simulink model "finalcode"  (R2020a)
settings: Solver=FixedStepDiscrete  StartTime=0.0  StopTime=1  FixedStep=0.0005  RelTol=1e-3  EnableMultiTasking=on
undefined symbols (not defined in the file): acc_calmax1, acc_calmax2, acc_calmin1, acc_calmin2, akemancanshu, angle_middle, bre, bre_calmax, bre_calmin, chasuniujvvvv_hou, chasuniujvvvv_qian, chasuuuu, ecucoder_acal, I_AN01_5K1, I_AN03_5V, I_AN04_5V, kd, kddd, ki, kiii, kp, kppp, leftmax, O_SW06_HS1A, P11111, P22222, PIDmodel, PPPP, rightmax, slip, slip_big, slip_little, slipmodel, T_add, T_del, tiaoshi, TTTTTyouren, vvvv, zhiling
libraries: ec5744lib x305, canmsglib x97, simulink x23
(part 8 of 11)

== system finalcode/Subsystem/Tx/转向/检查模式转向/Subsystem/Subsystem ==
  Enable : EnablePort
  CAN Pack : canmsglib/CAN Pack  CANdbFile=C:\Users\Liu keliang\Desktop\HRT2023\HRT23赛季刘科良\CANdbc\steering.dbc  MsgList=(none)  MsgName=enable123  MsgIDType=Standard (11-bit identifier)  MsgIdentifier=291  MsgLength=1  Remote=off  ApplyMinMax=off  BusOutput=off  SignalInfo={'enable123','0','8','LE','unsigned','Standard','0','1','0','0','255'}
      settings: SourceProductBaseCode=ME,XP,VN  DataFormat=CANdb specified signals
  CAN Pack1 : canmsglib/CAN Pack  CANdbFile=C:\Users\Liu keliang\Desktop\HRT2023\HRT23赛季刘科良\CANdbc\steering.dbc  MsgList=(none)  MsgName=enable0  MsgIDType=Standard (11-bit identifier)  MsgIdentifier=0  MsgLength=8  Remote=off  ApplyMinMax=off  BusOutput=off  SignalInfo={'enable_00','0','16','LE','unsigned','Standard','0','1','0','0','65535';'enable_00_Copy_1','16','16','LE','unsigned','Standard','0','1','0','0','65535';'enable_00_Copy_2','32','16','LE','unsigned','Standard','0','1','0','0','65535';'enable_00_Copy_3','48','16','LE','unsigned','Standard','0','1','0','0','65535'}
      settings: SourceProductBaseCode=ME,XP,VN  DataFormat=CANdb specified signals
  CAN Pack2 : canmsglib/CAN Pack  CANdbFile=C:\Users\Liu keliang\Desktop\HRT2023\HRT23赛季刘科良\CANdbc\steering.dbc  MsgList=(none)  MsgName=enable401  MsgIDType=Standard (11-bit identifier)  MsgIdentifier=1025  MsgLength=6  Remote=off  ApplyMinMax=off  BusOutput=off  SignalInfo={'enable401','0','8','LE','unsigned','Standard','0','1','0','0','255';'enable401_Copy_1','8','8','LE','unsigned','Standard','0','1','0','0','255';'enable401_Copy_2','16','32','LE','signed','Standard','0','1','0','-2147483648','2147483647'}
      settings: SourceProductBaseCode=ME,XP,VN  DataFormat=CANdb specified signals
  CAN Pack4 : canmsglib/CAN Pack  CANdbFile=C:\Users\Liu keliang\Desktop\HRT2023\HRT23赛季刘科良\CANdbc\steering.dbc  MsgList=(none)  MsgName=enable80  MsgIDType=Standard (11-bit identifier)  MsgIdentifier=128  MsgLength=1  Remote=off  ApplyMinMax=off  BusOutput=off  SignalInfo={'dingshi','0','8','LE','unsigned','Standard','0','1','0','0','255'}
      settings: SourceProductBaseCode=ME,XP,VN  DataFormat=CANdb specified signals
  CANPackMessage : ec5744lib/RapidECU_U4B/04CANCommunication/CANPackMessage  datalength=1  sampletime=-1
      settings: SourceProductName=ECUCoder for MPC5744
  CANPackMessage1 : ec5744lib/RapidECU_U4B/04CANCommunication/CANPackMessage  datalength=8  sampletime=-1
      settings: SourceProductName=ECUCoder for MPC5744
  CANPackMessage2 : ec5744lib/RapidECU_U4B/04CANCommunication/CANPackMessage  datalength=6  sampletime=-1
      settings: SourceProductName=ECUCoder for MPC5744
  CANPackMessage4 : ec5744lib/RapidECU_U4B/04CANCommunication/CANPackMessage  datalength=1  sampletime=-1
      settings: SourceProductName=ECUCoder for MPC5744
  CANTransmit : ec5744lib/RapidECU_U4B/04CANCommunication/CANTransmit  canmodule=2  canbuffer=15  canmessageid=hex2dec('123')  canmessagetype=Standard(11-bit ID)  datalength=1  sampletime=-1
      settings: SourceProductName=ECUCoder for MPC5744
  CANTransmit1 : ec5744lib/RapidECU_U4B/04CANCommunication/CANTransmit  canmodule=2  canbuffer=56  canmessageid=hex2dec('00')  canmessagetype=Standard(11-bit ID)  datalength=8  sampletime=-1
      settings: SourceProductName=ECUCoder for MPC5744
  CANTransmit2 : ec5744lib/RapidECU_U4B/04CANCommunication/CANTransmit  canmodule=2  canbuffer=57  canmessageid=hex2dec('401')  canmessagetype=Standard(11-bit ID)  datalength=6  sampletime=-1
      settings: SourceProductName=ECUCoder for MPC5744
  CANTransmit4 : ec5744lib/RapidECU_U4B/04CANCommunication/CANTransmit  canmodule=2  canbuffer=58  canmessageid=hex2dec('80')  canmessagetype=Standard(11-bit ID)  datalength=1  sampletime=-1
      settings: SourceProductName=ECUCoder for MPC5744
  Constant : Constant  Value=0  SampleTime=-1
  Constant1 : Constant  SampleTime=-1
  Constant{2..4,6} (4 alike) : Constant  Value=0
  Constant5 : Constant  Value=0  SampleTime=-1
  Data Type Conversion{,1..2,4} (4 alike) : DataTypeConversion  OutDataTypeStr=uint8
  MATLAB Function : MATLAB Function  TreatAsAtomicUnit=on
  Saturation : Saturate  UpperLimit=758000  LowerLimit=605000
  Terminator{,1..2,4} (4 alike) : Terminator
  Zero-Order Hold{,1..4} (5 alike) : ZeroOrderHold  SampleTime=-1
  wires:
  CANTransmit/1 -> Terminator/1
  Zero-Order Hold2/1 -> CAN Pack1/3
  MATLAB Function/2(y) -> CAN Pack2/1
  CAN Pack1/1 -> CANPackMessage1/1
  CANTransmit2/1 -> Terminator2/1
  CANPackMessage4/1 -> Data Type Conversion4/1
  CAN Pack2/1 -> CANPackMessage2/1
  CANTransmit1/1 -> Terminator1/1
  Constant/1 -> Zero-Order Hold/1
  Data Type Conversion1/1 -> CANTransmit1/1
  Constant6/1 -> CAN Pack2/2
  CANTransmit4/1 -> Terminator4/1
  Data Type Conversion/1 -> CANTransmit/1
  Zero-Order Hold/1 -> CAN Pack/1
  CANPackMessage2/1 -> Data Type Conversion2/1
  CANPackMessage/1 -> Data Type Conversion/1
  Data Type Conversion4/1 -> CANTransmit4/1
  Constant4/1 -> Zero-Order Hold3/1
  CAN Pack/1 -> CANPackMessage/1
  CANPackMessage1/1 -> Data Type Conversion1/1
  Constant5/1 -> Zero-Order Hold4/1
  CAN Pack4/1 -> CANPackMessage4/1
  Constant3/1 -> Zero-Order Hold2/1
  Constant2/1 -> Zero-Order Hold1/1
  Constant1/1 -> CAN Pack1/1
  Zero-Order Hold4/1 -> CAN Pack4/1
  MATLAB Function/1(steer) -> Saturation/1
  Zero-Order Hold1/1 -> CAN Pack1/2
  Data Type Conversion2/1 -> CANTransmit2/1
  Zero-Order Hold3/1 -> CAN Pack1/4
  Saturation/1 -> CAN Pack2/3

== system finalcode/Subsystem/Tx/转向/检查模式转向/Subsystem/Subsystem1 ==
  y1 : Inport
  y2 : Inport  Port=2
  Enable : EnablePort
  CAN Pack5 : canmsglib/CAN Pack  CANdbFile=C:\Users\Liu keliang\Desktop\HRT2023\HRT23赛季刘科良\CANdbc\zhuanxiangresetting.dbc  MsgList=(none)  MsgName=reseting  MsgIDType=Standard (11-bit identifier)  MsgIdentifier=1537  MsgLength=8  Remote=off  ApplyMinMax=off  BusOutput=off  SignalInfo={'reseting1','0','32','LE','unsigned','Standard','0','1','0','-Inf','Inf';'reseting2','32','32','LE','unsigned','Standard','0','1','0','-Inf','Inf'}
      settings: SourceProductBaseCode=ME,XP,VN  DataFormat=CANdb specified signals
  CANPackMessage3 : ec5744lib/RapidECU_U4B/04CANCommunication/CANPackMessage  datalength=8  sampletime=-1
      settings: SourceProductName=ECUCoder for MPC5744
  CANTransmit3 : ec5744lib/RapidECU_U4B/04CANCommunication/CANTransmit  canmodule=2  canbuffer=61  canmessageid=hex2dec('601')  canmessagetype=Standard(11-bit ID)  datalength=8  sampletime=-1
      settings: SourceProductName=ECUCoder for MPC5744
  Data Type Conversion3 : DataTypeConversion  OutDataTypeStr=uint8
  Terminator3 : Terminator
  wires:
  CAN Pack5/1 -> CANPackMessage3/1
  y1/1 -> CAN Pack5/1
  CANTransmit3/1 -> Terminator3/1
  Data Type Conversion3/1 -> CANTransmit3/1
  CANPackMessage3/1 -> Data Type Conversion3/1
  y2/1 -> CAN Pack5/2

== system finalcode/Subsystem/Tx/转向/转向换算/Subsystem/integral ==
  Data Store Read12 : DataStoreRead  DataStoreName=zhuanjiaobianmaqi
  Data Store Read13 : DataStoreRead  DataStoreName=workstation_steering
  Sum of Elements : Sum  Inputs=+
  Sum1 : Sum  Inputs=|-+
  Tapped Delay : simulink/Discrete/Tapped Delay  vinit=0.0  samptime=-1  NumDelays=20  DelayOrder=Oldest  includeCurrent=off
  Out1 : Outport
  wires:
  Data Store Read12/1 -> Sum1/1
  Data Store Read13/1 -> Sum1/2
  Sum of Elements/1 -> Out1/1
  Sum1/1 -> Tapped Delay/1
  Tapped Delay/1 -> Sum of Elements/1

== system finalcode/Subsystem/Tx/转向/转向换算/Subsystem/算术平均值滤波 ArithmeticAverage ==
  In1 : Inport
  Constant : Constant  Value=5
  Divide : Product  Inputs=*/
  Sum of Elements : Sum  Inputs=+
  Tapped Delay : simulink/Discrete/Tapped Delay  vinit=0.0  samptime=-1  NumDelays=5  DelayOrder=Oldest  includeCurrent=off
  Out1 : Outport
  wires:
  Tapped Delay/1 -> Sum of Elements/1
  In1/1 -> Tapped Delay/1
  Divide/1 -> Out1/1
  Sum of Elements/1 -> Divide/1
  Constant/1 -> Divide/2

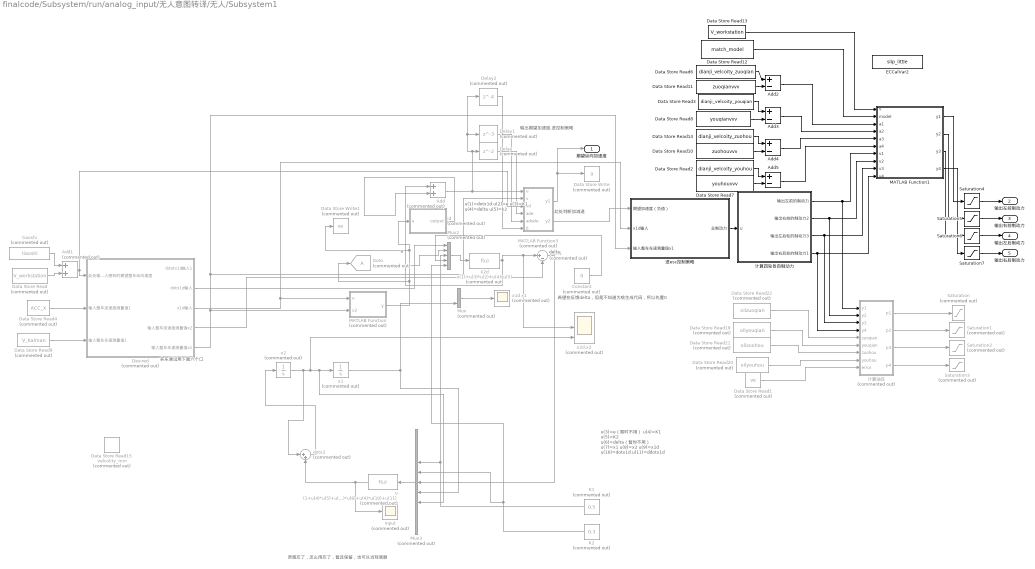
== system finalcode/Subsystem/run/analog_input/无人意图转译/无人/Subsystem1 ==
  note: 希望在反馈delta，但是不知道为啥生成代码，所以先置0
  note: 灵感忘了，怎么用忘了，暂且保留，也可以当观测器
  note: 输出期望加速度,进控制策略
  note: u(3)=e（暂时不用）
      | u(4)=K1
      | u(5)=K2
      | u(6)=delta（暂时不用）
      | u(7)=x1
      | u(8)=x2
      | u(9)=x1d
      | u(10)=dotx1d
      | u(11)=ddotx1d
  note: delta
  note: e
  note: 此处判断加减速
  note: 实车测试用下面六个口
  note: u(1)=dotx1d
      | u(2)=e
      | u(3)=K1
      | u(4)=delta
      | u(5)=k2
  Add : Sum  Commented=on
  Add1 : Sum  Commented=on
  Add{2..5} (4 alike) : Sum  Inputs=+-
  Constant : Constant  Commented=on  Value=0
  Data Store Read : DataStoreRead  Commented=on  DataStoreName=V_workstation
  Data Store Read1 : DataStoreRead  Commented=on  DataStoreName=ve
  Data Store Read10 : DataStoreRead  DataStoreName=zuohouvvv
  Data Store Read11 : DataStoreRead  DataStoreName=zuoqianvvv
  Data Store Read12 : DataStoreRead  DataStoreName=match_model
  Data Store Read13 : DataStoreRead  DataStoreName=V_workstation
  Data Store Read14 : DataStoreRead  DataStoreName=dianji_velcoity_zuohou
  Data Store Read15 : DataStoreRead  Commented=on  DataStoreName=velcolity_min
  Data Store Read19 : DataStoreRead  Commented=on  DataStoreName=oilyouqian
  Data Store Read2 : DataStoreRead  DataStoreName=dianji_velcoity_youhou
  Data Store Read20 : DataStoreRead  Commented=on  DataStoreName=oilyouhou
  Data Store Read21 : DataStoreRead  Commented=on  DataStoreName=oilzuohou
  Data Store Read22 : DataStoreRead  Commented=on  DataStoreName=oilzuoqian
  Data Store Read3 : DataStoreRead  DataStoreName=dianji_velcoity_youqian
  Data Store Read4 : DataStoreRead  Commented=on  DataStoreName=ACC_X
  Data Store Read6 : DataStoreRead  DataStoreName=dianji_velcoity_zuoqian
  Data Store Read7 : DataStoreRead  DataStoreName=youhouvvv
  Data Store Read8 : DataStoreRead  DataStoreName=youqianvvv
  Data Store Read9 : DataStoreRead  Commented=on  DataStoreName=V_Kalman
  Data Store Write : DataStoreWrite  Commented=on  DataStoreName=a
  Data Store Write1 : DataStoreWrite  Commented=on  DataStoreName=ve
  Delay : Delay  Commented=on
  Delay1 : Delay  Commented=on  DelayLength=3
  Delay2 : Delay  Commented=on  DelayLength=4
  Desired : Subsystem  Commented=on
  ECCalVar2 : Constant  InitFcn=ecucoder_acal;  Value=slip_little  OutDataTypeStr=Inherit: Inherit via back propagation  SampleTime=-1
  Goto : Goto  Commented=on  TagVisibility=global
  "Input " : Scope  Commented=on
  K1 : Constant  Commented=on  Value=0.5
  K2 : Constant  Commented=on  Value=0.3
  MATLAB Function : MATLAB Function  Commented=on  TreatAsAtomicUnit=on
  MATLAB Function1 : MATLAB Function  TreatAsAtomicUnit=on
  MATLAB Function3 : MATLAB Function  Commented=on  TreatAsAtomicUnit=on
  Mux : Mux  Commented=on  Inputs=2
  Mux2 : Mux  Commented=on  Inputs=5
  Mux3 : Mux  Commented=on  Inputs=11
  Saturation{,1..3} (4 alike) : Saturate  Commented=on  UpperLimit=4500  LowerLimit=0
  Saturation{4..7} (4 alike) : Saturate  UpperLimit=2100  LowerLimit=0
  Sum1 : Sum  Commented=on  Inputs=|+-
  X2d : Fcn  Commented=on  Expr=u(1)+u(3)*u(2)+u(4)*u(5)
  dotx2 : Sum  Commented=on  Inputs=|++
  id : MATLAB Function  Commented=on  TreatAsAtomicUnit=on
  tiaoshi : Constant  Commented=on  InitFcn=ecucoder_acal;  Value=tiaoshi  OutDataTypeStr=double  SampleTime=-1
  u : Fcn  Commented=on  Expr=(1+u(4)*u(5)+u(5))*u(9)-(1+u(4)*u(5))*u(7)-(u(4)+u(5)-1)*u(8)+u(4)*u(10)+u(11)
  x1 : Integrator  Commented=on
  x1d x1 : Scope  Commented=on
  x2 : Integrator  Commented=on  UpperSaturationLimit=10  ZeroCross=off
  x2d,x2 : Scope  Commented=on  NumInputPorts=3
  计算四轮各自制动力 : Subsystem
  计算油压 : MATLAB Function  Commented=on  TreatAsAtomicUnit=on
  进esc控制策略 : Subsystem
  期望纵向加速度 : Outport
  输出左前制动力 : Outport  Port=2
  输出右前制动力 : Outport  Port=3
  输出左后制动力 : Outport  Port=4
  输出右后制动力 : Outport  Port=5
  wires:
  K2/1 -> Mux2/5, Mux3/5
  计算油压/1(p1) -> Saturation/1
  MATLAB Function/1(y) -> id/1(u), Data Store Write1/1, Mux2/2, Goto/1
  Desired/4(输入整车加速度测量值x2) -> Sum1/2
  x2/1 -> dotx2/1, x2d,x2/3, x1/1, Mux3/8
  Sum1/1 -> Mux3/6
  计算油压/2(p2) -> Saturation1/1
  MATLAB Function3/2(y2) -> 进esc控制策略/1(期望加速度（负值）)
  计算四轮各自制动力/1(输出左前的制动力) -> MATLAB Function1/7(v1), 计算油压/1(y1)
  Mux/1 -> x1d x1/1
  u/1 -> dotx2/2, "Input "/1
  计算油压/3(p3) -> Saturation2/1
  计算四轮各自制动力/3(输出左后轮的制动力3) -> MATLAB Function1/9(v3), 计算油压/3(y3)
  计算油压/4(p4) -> Saturation3/1
  计算四轮各自制动力/4(输出右后轮的制动力1) -> MATLAB Function1/10(v4), 计算油压/4(y4)
  进esc控制策略/1(总制动力) -> 计算四轮各自制动力/1(u)
  K1/1 -> Mux2/3, Mux3/4
  dotx2/1 -> x2/1
  Mux2/1 -> X2d/1
  Mux3/1 -> u/1
  x1/1 -> Mux/2, Mux3/7
  Data Store Read9/1 -> Desired/3(输入整车车速测量值1)
  Data Store Read4/1 -> Desired/2(输入整车加速度测量值1)
  X2d/1 -> x2d,x2/2, Sum1/1, Add/1
  Constant/1 -> Mux2/4
  MATLAB Function3/1(y1) -> Data Store Write/1, 期望纵向加速度/1
  Desired/3(x1d输入) -> 进esc控制策略/2(x1d输入), MATLAB Function/1(u)
  Desired/2(dotx1d输入) -> Mux2/1
  tiaoshi/1 -> Add1/1
  Data Store Read/1 -> Add1/2
  Add1/1 -> Desired/1(此处输入感知的期望整车纵向速度), MATLAB Function3/3(vd)
  Desired/5(输入整车车速测量值x1) -> 进esc控制策略/3(输入整车车速测量值x1), MATLAB Function3/2(v), MATLAB Function/2(u2)
  Add/1 -> Delay1/1, Delay2/1, Delay/1, MATLAB Function3/1(u)
  Delay/1 -> MATLAB Function3/4(ade)
  Delay1/1 -> MATLAB Function3/5(adede)
  Delay2/1 -> MATLAB Function3/6(adedede)
  id/1(output) -> Add/2
  Data Store Read20/1 -> 计算油压/8(youhou)
  Data Store Read21/1 -> 计算油压/7(zuohou)
  Data Store Read22/1 -> 计算油压/5(zuoqian)
  Data Store Read19/1 -> 计算油压/6(youqian)
  Data Store Read1/1 -> 计算油压/9(error)
  计算四轮各自制动力/2(输出右前的制动力2) -> 计算油压/2(y2), MATLAB Function1/8(v2)
  Saturation4/1 -> 输出左前制动力/1
  Saturation5/1 -> 输出右前制动力/1
  Saturation6/1 -> 输出左后制动力/1
  Saturation7/1 -> 输出右后制动力/1
  Data Store Read11/1 -> Add2/2
  Data Store Read6/1 -> Add2/1
  Data Store Read8/1 -> Add3/2
  Data Store Read3/1 -> Add3/1
  Data Store Read14/1 -> Add4/1
  Data Store Read10/1 -> Add4/2
  Data Store Read7/1 -> Add5/2
  Data Store Read2/1 -> Add5/1
  Data Store Read13/1 -> MATLAB Function1/1(v)
  Data Store Read12/1 -> MATLAB Function1/2(model)
  Add2/1 -> MATLAB Function1/3(a1)
  Add3/1 -> MATLAB Function1/4(a2)
  Add4/1 -> MATLAB Function1/5(a3)
  Add5/1 -> MATLAB Function1/6(a4)
  MATLAB Function1/1(y1) -> Saturation4/1
  MATLAB Function1/2(y2) -> Saturation5/1
  MATLAB Function1/3(y3) -> Saturation6/1
  MATLAB Function1/4(y4) -> Saturation7/1

== system finalcode/Subsystem/run/analog_input/有人/扭矩分配/Enabled Subsystem ==
  Constant : Constant  Value=1.18
  Constant1 : Constant  Value=0.7
  Data Store Read : DataStoreRead  DataStoreName=dianji_velcoity_zuoqian
  Data Store Read1 : DataStoreRead  DataStoreName=dianji_velcoity_youhou
  Data Store Read10 : DataStoreRead  DataStoreName=shucai_ay
  Data Store Read11 : DataStoreRead  DataStoreName=zhuanjiaobianmaqi
  Data Store Read3 : DataStoreRead  DataStoreName=shucai_ay
  Data Store Read4 : DataStoreRead  DataStoreName=dianji_velcoity_youqian
  Data Store Read5 : DataStoreRead  DataStoreName=dianji_velcoity_zuohou
  Data Store Read6 : DataStoreRead  DataStoreName=shucai_az
  Data Store Read7 : DataStoreRead  DataStoreName=V_Kalman
  Data Store Read8 : DataStoreRead  DataStoreName=zhuanjiaobianmaqi
  Data Store Read9 : DataStoreRead  DataStoreName=V_Kalman
  Delay : Delay  DelayLength=1
  Delay1 : Delay  DelayLength=1
  LQR差速 : MATLAB Function  TreatAsAtomicUnit=on
  MATLAB Function1 : MATLAB Function  TreatAsAtomicUnit=on
  MATLAB Function2 : MATLAB Function  TreatAsAtomicUnit=on
  Product2 : Product
  Sum : Sum  Inputs=|+-
  kalman_filter : MATLAB Function  TreatAsAtomicUnit=on
  期望横摆力矩计算 : MATLAB Function  TreatAsAtomicUnit=on
  横摆角速度 : MATLAB Function  TreatAsAtomicUnit=on
  转动惯量1 : Constant  Value=145
  y : Outport
  wires:
  Constant1/1 -> 横摆角速度/9(k)
  横摆角速度/2(wz2) -> kalman_filter/4(w_z2)
  Product2/1 -> Sum/2
  期望横摆力矩计算/1(Mz) -> Sum/1
  转动惯量1/1 -> LQR差速/3(J), Product2/1
  Data Store Read8/1 -> 横摆角速度/8(alpha)
  Data Store Read7/1 -> 横摆角速度/2(vx)
  Data Store Read6/1 -> Product2/2, LQR差速/2(yaw_rate)
  Sum/1 -> LQR差速/1(yaw_error)
  Constant/1 -> 横摆角速度/7(Bf)
  Delay/1 -> kalman_filter/2(w_k_1)
  Data Store Read/1 -> 横摆角速度/4(vfl)
  Data Store Read5/1 -> 横摆角速度/5(vrl)
  kalman_filter/1(y) -> 期望横摆力矩计算/1(delta)
  Data Store Read1/1 -> 横摆角速度/6(vrr)
  Data Store Read3/1 -> 横摆角速度/1(ay)
  LQR差速/1(M) -> MATLAB Function2/2(M)  "附加"
  Data Store Read9/1 -> 期望横摆力矩计算/2(Vx)
  Data Store Read10/1 -> 期望横摆力矩计算/3(ax)
  Data Store Read4/1 -> 横摆角速度/3(vfr)
  MATLAB Function1/1(az) -> Delay1/1
  横摆角速度/1(wz1) -> MATLAB Function1/1(w_z), Delay/1, kalman_filter/3(w_k)
  Delay1/1 -> kalman_filter/1(a_k_1)
  Data Store Read11/1 -> MATLAB Function2/1(angle)
  MATLAB Function2/1(y) -> y/1

== system finalcode/Subsystem/run/analog_input/有人/踏板标定/Subsystem ==
  Enable : EnablePort
  Data Type Conversion{,1,4..7} (6 alike) : DataTypeConversion  OutDataTypeStr=single
  ECCalVar1 : Constant  InitFcn=ecucoder_acal;  Value=acc_calmax1  OutDataTypeStr=double  SampleTime=-1
  ECCalVar2 : Constant  InitFcn=ecucoder_acal;  Value=acc_calmin1  OutDataTypeStr=double  SampleTime=-1
  ECCalVar3 : Constant  InitFcn=ecucoder_acal;  Value=acc_calmax2  OutDataTypeStr=double  SampleTime=-1
  ECCalVar4 : Constant  InitFcn=ecucoder_acal;  Value=acc_calmin2  OutDataTypeStr=double  SampleTime=-1
  ECCalVar5 : Constant  InitFcn=ecucoder_acal;  Value=bre_calmax  OutDataTypeStr=double  SampleTime=-1
  ECCalVar6 : Constant  InitFcn=ecucoder_acal;  Value=bre_calmin  OutDataTypeStr=double  SampleTime=-1
  FRAMEnable : ec5744lib/RapidECU_U4B/12EEModule/FRAMEnable  framenable=off
      settings: SourceProductName=ECUCoder for MPC5744
  FRAMWrite1 : ec5744lib/RapidECU_U4B/12EEModule/FRAMWrite  buffer=6  sampletime=-1
      settings: SourceProductName=ECUCoder for MPC5744
  FRAMWrite2 : ec5744lib/RapidECU_U4B/12EEModule/FRAMWrite  buffer=4  sampletime=-1
      settings: SourceProductName=ECUCoder for MPC5744
  FRAMWrite3 : ec5744lib/RapidECU_U4B/12EEModule/FRAMWrite  buffer=5  sampletime=-1
      settings: SourceProductName=ECUCoder for MPC5744
  FRAMWrite4 : ec5744lib/RapidECU_U4B/12EEModule/FRAMWrite  buffer=7  sampletime=-1
      settings: SourceProductName=ECUCoder for MPC5744
  FRAMWrite5 : ec5744lib/RapidECU_U4B/12EEModule/FRAMWrite  buffer=8  sampletime=-1
      settings: SourceProductName=ECUCoder for MPC5744
  FRAMWrite6 : ec5744lib/RapidECU_U4B/12EEModule/FRAMWrite  buffer=9  sampletime=-1
      settings: SourceProductName=ECUCoder for MPC5744
  wires:
  ECCalVar2/1 -> Data Type Conversion/1
  Data Type Conversion/1 -> FRAMWrite5/1
  ECCalVar5/1 -> Data Type Conversion7/1
  Data Type Conversion7/1 -> FRAMWrite3/1
  Data Type Conversion6/1 -> FRAMWrite2/1
  ECCalVar6/1 -> Data Type Conversion6/1
  ECCalVar3/1 -> Data Type Conversion5/1
  Data Type Conversion5/1 -> FRAMWrite4/1
  ECCalVar4/1 -> Data Type Conversion4/1
  Data Type Conversion4/1 -> FRAMWrite1/1
  ECCalVar1/1 -> Data Type Conversion1/1
  Data Type Conversion1/1 -> FRAMWrite6/1

== system finalcode/Subsystem/run/analog_input/有人/踏板标定/Subsystem1 ==
  ECCalVar1 : Constant  InitFcn=ecucoder_acal;  Value=acc_calmax1  OutDataTypeStr=double  SampleTime=-1
  ECCalVar2 : Constant  InitFcn=ecucoder_acal;  Value=acc_calmin1  OutDataTypeStr=double  SampleTime=-1
  ECCalVar3 : Constant  InitFcn=ecucoder_acal;  Value=acc_calmax2  OutDataTypeStr=double  SampleTime=-1
  ECCalVar4 : Constant  InitFcn=ecucoder_acal;  Value=acc_calmin2  OutDataTypeStr=double  SampleTime=-1
  ECCalVar5 : Constant  InitFcn=ecucoder_acal;  Value=bre_calmax  OutDataTypeStr=double  SampleTime=-1
  ECCalVar6 : Constant  InitFcn=ecucoder_acal;  Value=bre_calmin  OutDataTypeStr=double  SampleTime=-1
  MATLAB Function : MATLAB Function  TreatAsAtomicUnit=on
  Max : MinMax  Function=max  Inputs=6
  y : Outport
  wires:
  ECCalVar3/1 -> Max/4
  ECCalVar2/1 -> Max/1
  ECCalVar4/1 -> Max/3
  ECCalVar5/1 -> Max/6
  ECCalVar1/1 -> Max/2
  ECCalVar6/1 -> Max/5
  Max/1 -> MATLAB Function/1(u)
  MATLAB Function/1(y) -> y/1

== system finalcode/Subsystem/run/analog_input/有人/踏板标定/算术平均值滤波 ArithmeticAverage1 ==
  In1 : Inport
  Constant : Constant  Value=5
  Divide : Product  Inputs=*/
  Sum of Elements : Sum  Inputs=+
  Tapped Delay : simulink/Discrete/Tapped Delay  vinit=0.0  samptime=-1  NumDelays=5  DelayOrder=Oldest  includeCurrent=off
  angle : Outport
  wires:
  Tapped Delay/1 -> Sum of Elements/1
  In1/1 -> Tapped Delay/1
  Divide/1 -> angle/1
  Sum of Elements/1 -> Divide/1
  Constant/1 -> Divide/2

== system finalcode/Subsystem/run/analog_input/有人/限滑/Enabled Subsystem ==
  note: 转动惯量系数
      | 加速度大小参数
  zuoqian : Inport
  youqian : Inport  Port=2
  zuohou : Inport  Port=3
  youhou : Inport  Port=4
  Constant{,1..3} (4 alike) : Constant  Value=0.9
  Data Store Read : DataStoreRead  DataStoreName=slipzuoqian
  Data Store Read1 : DataStoreRead  DataStoreName=slipzuohou
  Data Store Read2 : DataStoreRead  DataStoreName=slipyuoqian
  Data Store Read3 : DataStoreRead  DataStoreName=slipyouhou
  Data Store Read4 : DataStoreRead  Commented=on  DataStoreName=V_Kalman
  MATLAB Function : MATLAB Function  Commented=on  TreatAsAtomicUnit=on
  MATLAB Function1 : MATLAB Function  Commented=on  TreatAsAtomicUnit=on
  pid限滑 : MATLAB Function  TreatAsAtomicUnit=on
  pid限滑1 : MATLAB Function  TreatAsAtomicUnit=on
  pid限滑2 : MATLAB Function  TreatAsAtomicUnit=on
  pid限滑3 : MATLAB Function  TreatAsAtomicUnit=on
  M_zuoqian : Outport
  M_youqian : Outport  Port=2
  M_zuohou : Outport  Port=3
  M_youhou : Outport  Port=4
  wires:
  Data Store Read/1 -> pid限滑/1(slip)
  Constant/1 -> pid限滑/2(slip_ratio_limit)
  pid限滑1/1(M) -> M_youqian/1
  zuoqian/1 -> pid限滑/3(u)
  Data Store Read3/1 -> pid限滑3/1(slip)
  pid限滑2/1(M) -> M_zuohou/1
  pid限滑3/1(M) -> M_youhou/1
  Constant1/1 -> pid限滑1/2(slip_ratio_limit)
  Constant2/1 -> pid限滑2/2(slip_ratio_limit)
  Data Store Read1/1 -> pid限滑2/1(slip)
  zuohou/1 -> pid限滑2/3(u)
  Constant3/1 -> pid限滑3/2(slip_ratio_limit)
  youhou/1 -> pid限滑3/3(u)
  youqian/1 -> pid限滑1/3(u)
  Data Store Read2/1 -> pid限滑1/1(slip)
  MATLAB Function/1(M) -> MATLAB Function1/1(u1)
  Data Store Read4/1 -> MATLAB Function/1(v)
  pid限滑/1(M) -> M_zuoqian/1

== system finalcode/Subsystem/run/analog_input/有人/限滑/Enabled Subsystem1 ==
  zuoqian : Inport
  youqian : Inport  Port=2
  zuohou : Inport  Port=3
  youhou : Inport  Port=4
  M_zuoqian : Outport
  M_youqian : Outport  Port=2
  M_zuohou : Outport  Port=3
  M_youhou : Outport  Port=4
  wires:
  zuoqian/1 -> M_zuoqian/1
  zuohou/1 -> M_zuohou/1
  youqian/1 -> M_youqian/1
  youhou/1 -> M_youhou/1

== system finalcode/Subsystem/run/ctrl/Subsystem1/control_strategy/Subsystem ==
  alpha : Inport
  beta : Inport  Port=2
  -1~1 : Saturate  Commented=on  UpperLimit=1  LowerLimit=-1
  0~5 : Saturate  Commented=on  UpperLimit=5  LowerLimit=0
  Mux : Mux  Commented=on  Inputs=3
  Mux1 : Mux  Commented=on  Inputs=5
  Mux2 : Mux  Commented=on  Inputs=5
  Rules : Subsystem  Commented=on
  Scope alpha : Scope  Commented=on
  Scope beta : Scope  Commented=on
  Scope delta : Scope  Commented=on
  Scope delta sets : Scope  Commented=on
  a1 : Constant  Commented=on  Value=1.2
  a2 : Constant  Commented=on  Value=2.4
  alpha test : simulink/Sources/Ramp  Commented=on  slope=0.1  start=0  InitialOutput=-0.5
  b1 : Constant  Commented=on  Value=-0.5
  b2 : Constant  Commented=on  Value=0
  b3 : Constant  Commented=on  Value=0.5
  beta test : simulink/Sources/Ramp  Commented=on  slope=0.1  start=0  InitialOutput=-1.5
  d1 : Constant  Commented=on  Value=-0.5
  d2 : Constant  Commented=on  Value=0
  d3 : Constant  Commented=on  Value=0.5
  defuzzification : MATLAB Function  Commented=on  TreatAsAtomicUnit=on
  α sets : MATLAB Function  Commented=on  TreatAsAtomicUnit=on
  β sets : MATLAB Function  Commented=on  TreatAsAtomicUnit=on
  delta : Outport  VectorParamsAs1DForOutWhenUnconnected=off
  wires:
  defuzzification/1(delta) -> delta/1, Scope delta/1  "delta"
  Rules/3(do) -> Mux2/3, defuzzification/3(do)
  Rules/5(dpb) -> Mux2/5, defuzzification/5(dpb)
  beta/1 -> -1~1/1
  b3/1 -> β sets/4(b3)
  α sets/1(as) -> Mux/1, Rules/1(as)  "as"
  β sets/3(bo) -> Mux1/3, Rules/6(bo)  "bo"
  d2/1 -> defuzzification/7(d2)
  Rules/4(dps) -> Mux2/4, defuzzification/4(dps)
  β sets/1(bnb) -> Mux1/1, Rules/4(bnb)  "bnb"
  Rules/2(dns) -> Mux2/2, defuzzification/2(dns)
  Mux/1 -> Scope alpha/1
  d1/1 -> defuzzification/6(d1)
  Mux2/1 -> Scope delta sets/1
  β sets/2(bns) -> Mux1/2, Rules/5(bns)  "bns"
  β sets/5(bpb) -> Mux1/5, Rules/8(bpb)  "bpb"
  0~5/1 -> α sets/1(alpha)
  a1/1 -> α sets/2(a1)
  alpha/1 -> 0~5/1
  β sets/4(bps) -> Mux1/4, Rules/7(bps)  "bps"
  Rules/1(dnb) -> Mux2/1, defuzzification/1(dnb)
  Mux1/1 -> Scope beta/1
  -1~1/1 -> β sets/1(beta)
  b2/1 -> β sets/3(b2)
  b1/1 -> β sets/2(b1)
  a2/1 -> α sets/3(a2)
  α sets/2(am) -> Mux/2, Rules/2(am)
  d3/1 -> defuzzification/8(d3)
  α sets/3(ab) -> Mux/3, Rules/3(ab)  "ab"

== system finalcode/Subsystem/run/ctrl/Subsystem1/control_strategy/差速 ==
  u : Inport
  Enable : EnablePort
  MATLAB Function3 : MATLAB Function  TreatAsAtomicUnit=on
  差速 : Subsystem
  youhou : Outport
  youqian : Outport  Port=2
  zuohou : Outport  Port=3
  zuoqian : Outport  Port=4
  wires:
  MATLAB Function3/3(zuohou) -> zuohou/1
  MATLAB Function3/4(zuoqian) -> zuoqian/1
  差速/1(M) -> MATLAB Function3/2(M)
  MATLAB Function3/2(youqian) -> youqian/1
  u/1 -> MATLAB Function3/1(u)
  MATLAB Function3/1(youhou) -> youhou/1

== system finalcode/Subsystem/run/ctrl/Subsystem1/control_strategy/限滑 ==
  In1 : Inport
  MATLAB Function : MATLAB Function  Commented=on  TreatAsAtomicUnit=on
  MPC : Subsystem
  PID限滑 : Subsystem
  Subsystem1 : Subsystem
  youhou : Outport
  youqian : Outport  Port=2
  zuohou : Outport  Port=3
  zuoqian : Outport  Port=4
  wires:
  MPC/2(左后) -> Subsystem1/8(mpc)
  PID限滑/2(throttle_youqian) -> Subsystem1/6(throttle_youqian)
  In1/1 -> PID限滑/1(u), Subsystem1/10(In7), MPC/4(左前in), Subsystem1/1(TP), MPC/1(右后in), Subsystem1/7(u), MPC/2(左后in), Subsystem1/4(In4), MPC/3(右前in)
  MPC/3(右前) -> Subsystem1/5(右前)
  PID限滑/4(throttle_zuoqian) -> Subsystem1/12(throttle_zuoqian)
  PID限滑/3(throttle_zuohou) -> Subsystem1/9(pid)
  MPC/1(右后) -> Subsystem1/2(右后)
  MPC/4(左前) -> Subsystem1/11(左前)
  PID限滑/1(throttle_youhou) -> Subsystem1/3(throttle_youhou)
  Subsystem1/1(youhou) -> youhou/1
  Subsystem1/4(zuoqian) -> zuoqian/1
  Subsystem1/3(zuohou) -> zuohou/1
  Subsystem1/2(youqian) -> youqian/1

== system finalcode/Subsystem/run/analog_input/无人意图转译/无人/Subsystem1/Desired ==
  此处输入感知的期望整车纵向速度 : Inport
  输入整车加速度测量值1 : Inport  Port=2
  输入整车车速测量值1 : Inport  Port=3
  Data Store Read3 : DataStoreRead  DataStoreName=match_model
  Data Store Write : DataStoreWrite  Commented=on  DataStoreName=acc
  MATLAB Function : MATLAB Function  TreatAsAtomicUnit=on
  MATLAB Function1 : MATLAB Function  Commented=on  TreatAsAtomicUnit=on
  MATLAB Function2 : MATLAB Function  TreatAsAtomicUnit=on
  Subsystem : Subsystem
  Subsystem1 : Subsystem
  ddotx1d输入1 : Outport
  dotx1d输入 : Outport  Port=2
  x1d输入 : Outport  Port=3
  输入整车加速度测量值x2 : Outport  Port=4
  输入整车车速测量值x1 : Outport  Port=5
  wires:
  此处输入感知的期望整车纵向速度/1 -> MATLAB Function2/7(v1), Subsystem1/1(y), MATLAB Function/1(u)
  输入整车加速度测量值1/1 -> 输入整车加速度测量值x2/1
  MATLAB Function1/1(y) -> ddotx1d输入1/1
  MATLAB Function/1(y) -> MATLAB Function2/1(u1), Subsystem/1(y)
  MATLAB Function2/1(y) -> MATLAB Function1/1(u), dotx1d输入/1, Data Store Write/1
  Subsystem/1(u2) -> MATLAB Function2/2(u2)
  Subsystem/2(u3) -> MATLAB Function2/3(u3)
  Subsystem/3(u4) -> MATLAB Function2/4(u4)
  Subsystem/4(u5) -> MATLAB Function2/5(u5)
  输入整车车速测量值1/1 -> 输入整车车速测量值x1/1
  Data Store Read3/1 -> MATLAB Function2/6(model)
  Subsystem1/1(u2) -> MATLAB Function2/8(v2)
  Subsystem1/2(u3) -> MATLAB Function2/9(v3)
  Subsystem1/3(u4) -> MATLAB Function2/10(v4)
  Subsystem1/4(u5) -> MATLAB Function2/11(v5)
  MATLAB Function2/2(V) -> x1d输入/1

== system finalcode/Subsystem/run/analog_input/无人意图转译/无人/Subsystem1/计算四轮各自制动力 ==
  u : Inport
  Data Store Read : DataStoreRead  DataStoreName=M_expire
  MATLAB Function : MATLAB Function  TreatAsAtomicUnit=on
  MeaModule : ec5744lib/RapidECU_U4B/07Calibration/MeaModule  signal=NT2
      settings: SourceProductName=ECUCoder for MPC5744
  输出左前的制动力 : Outport
  输出右前的制动力2 : Outport  Port=2
  输出左后轮的制动力3 : Outport  Port=3
  输出右后轮的制动力1 : Outport  Port=4
  wires:
  u/1 -> MATLAB Function/1(u)
  MATLAB Function/1(y1) -> MeaModule/1
  MATLAB Function/2(y2) -> 输出右前的制动力2/1
  MATLAB Function/3(y3) -> 输出左后轮的制动力3/1
  MATLAB Function/4(y4) -> 输出右后轮的制动力1/1
  Data Store Read/1 -> MATLAB Function/2(deltaM)
  MeaModule/1 -> 输出左前的制动力/1

== system finalcode/Subsystem/run/analog_input/无人意图转译/无人/Subsystem1/进esc控制策略 ==
  note: 反馈系数，得调一下
  期望加速度（负值） : Inport
  x1d输入 : Inport  Port=2
  输入整车车速测量值x1 : Inport  Port=3
  Abs : Abs
  Abs1 : Abs  Commented=on
  Data Store Read : DataStoreRead  DataStoreName=V_workstation
  Data Store Read9 : DataStoreRead  DataStoreName=V_Kalman
  MATLAB Function : MATLAB Function  Commented=on  TreatAsAtomicUnit=on
  MATLAB Function1 : MATLAB Function  Commented=on  TreatAsAtomicUnit=on
  MATLAB Function2 : MATLAB Function  TreatAsAtomicUnit=on
  MATLAB Function3 : MATLAB Function  TreatAsAtomicUnit=on
  MeaModule : ec5744lib/RapidECU_U4B/07Calibration/MeaModule  signal=NT1
      settings: SourceProductName=ECUCoder for MPC5744
  Product : Product
  Sum : Sum  Inputs=|++
  e : From  Commented=on  TagVisibility=global
  integral : MATLAB Function  Commented=on  TreatAsAtomicUnit=on
  pid_function : Subsystem  Commented=on
  整车质量 : Constant  Value=247
  总制动力 : Outport
  wires:
  Abs/1 -> Product/2
  整车质量/1 -> Product/1
  Product/1 -> Sum/1
  e/1 -> pid_function/1(u)
  pid_function/1(output) -> Abs1/1
  Abs1/1 -> Sum/2
  Sum/1 -> MeaModule/1, MATLAB Function/1(u), MATLAB Function1/2(u)
  输入整车车速测量值x1/1 -> MATLAB Function/2(v), MATLAB Function1/3(v), integral/1(u)
  x1d输入/1 -> integral/2(vd), MATLAB Function1/4(vd), MATLAB Function/3(vd)
  integral/1(output) -> MATLAB Function1/1(output)
  Data Store Read9/1 -> MATLAB Function3/2(v_k)
  期望加速度（负值）/1 -> pid_function/2(期望加速度（负值）)
  MATLAB Function3/1(y) -> Abs/1
  MeaModule/1 -> 总制动力/1
  Data Store Read/1 -> MATLAB Function3/1(v)

== system finalcode/Subsystem/run/ctrl/Subsystem1/control_strategy/Subsystem/Rules ==
  as : Inport
  am : Inport  Port=2
  ab : Inport  Port=3
  bnb : Inport  Port=4
  bns : Inport  Port=5
  bo : Inport  Port=6
  bps : Inport  Port=7
  bpb : Inport  Port=8
  DNB : MinMax  Function=max
  DNS : MinMax  Function=max  Inputs=3
  DO : MinMax  Function=max  Inputs=3
  DPB : MinMax  Function=max  Inputs=4
  DPS : MinMax  Function=max  Inputs=4
  Min(AB,BNB) : MinMax  Inputs=2
  Min(AB,BNS) : MinMax  Inputs=2
  Min(AB,BO) : MinMax  Inputs=2
  Min(AB,BPB) : MinMax  Inputs=2
  Min(AB,BPS) : MinMax  Inputs=2
  Min(AM,BNB) : MinMax  Inputs=2
  Min(AM,BNS) : MinMax  Inputs=2
  Min(AM,BO) : MinMax  Inputs=2
  Min(AM,BPB) : MinMax  Inputs=2
  Min(AM,BPS) : MinMax  Inputs=2
  Min(AS,BNB) : MinMax  Inputs=2
  Min(AS,BNS) : MinMax  Inputs=2
  Min(AS,BO) : MinMax  Inputs=2
  Min(AS,BPB) : MinMax  Inputs=2
  Min(AS,BPS) : MinMax  Inputs=2
  dnb : Outport  VectorParamsAs1DForOutWhenUnconnected=off
  dns : Outport  Port=2  VectorParamsAs1DForOutWhenUnconnected=off
  do : Outport  Port=3  VectorParamsAs1DForOutWhenUnconnected=off
  dps : Outport  Port=4  VectorParamsAs1DForOutWhenUnconnected=off
  dpb : Outport  Port=5  VectorParamsAs1DForOutWhenUnconnected=off
  wires:
  Min(AS,BNS)/1 -> DNS/1
  Min(AB,BNB)/1 -> DNS/3
  bps/1 -> Min(AB,BPS)/2, Min(AM,BPS)/2, Min(AS,BPS)/2
  bo/1 -> Min(AB,BO)/2, Min(AM,BO)/2, Min(AS,BO)/2
  bpb/1 -> Min(AB,BPB)/2, Min(AM,BPB)/2, Min(AS,BPB)/2
  as/1 -> Min(AS,BPB)/1, Min(AS,BPS)/1, Min(AS,BO)/1, Min(AS,BNS)/1, Min(AS,BNB)/1
  Min(AS,BNB)/1 -> DNB/1
  Min(AS,BPB)/1 -> DPB/1
  bns/1 -> Min(AB,BNS)/2, Min(AM,BNS)/2, Min(AS,BNS)/2
  Min(AB,BNS)/1 -> DO/3
  ab/1 -> Min(AB,BPB)/1, Min(AB,BPS)/1, Min(AB,BO)/1, Min(AB,BNS)/1, Min(AB,BNB)/1
  bnb/1 -> Min(AM,BNB)/2, Min(AS,BNB)/2, Min(AB,BNB)/2
  Min(AM,BO)/1 -> DPS/3
  am/1 -> Min(AM,BPB)/1, Min(AM,BPS)/1, Min(AM,BO)/1, Min(AM,BNS)/1, Min(AM,BNB)/1
  Min(AB,BPB)/1 -> DPB/3
  Min(AM,BNB)/1 -> DNS/2
  Min(AS,BPS)/1 -> DPS/1
  Min(AM,BPS)/1 -> DPS/2
  Min(AM,BNS)/1 -> DO/2
  Min(AB,BO)/1 -> DPS/4
  Min(AS,BO)/1 -> DO/1
  Min(AM,BPB)/1 -> DPB/2
  Min(AB,BPS)/1 -> DPB/4
  DO/1 -> do/1
  DNB/1 -> dnb/1
  DNS/1 -> dns/1
  DPS/1 -> dps/1
  DPB/1 -> dpb/1

== system finalcode/Subsystem/run/ctrl/Subsystem1/control_strategy/差速/差速 ==
  note: *待更改
  Data Store Read : DataStoreRead  DataStoreName=workstation_steering
  Data Store Read1 : DataStoreRead  DataStoreName=V_Kalman
  Data Store Read2 : DataStoreRead  DataStoreName=A_cexiang
  Data Store Read3 : DataStoreRead  DataStoreName=ACC_Z
  Data Store Read4 : DataStoreRead  Commented=on  DataStoreName=dianji_velcoity_zuoqian
  Data Store Read5 : DataStoreRead  Commented=on  DataStoreName=dianji_velcoity_youqian
  Data Store Read6 : DataStoreRead  Commented=on  DataStoreName=dianji_velcoity_zuohou
  Data Store Read7 : DataStoreRead  Commented=on  DataStoreName=dianji_velcoity_youhou
  Data Store Read8 : DataStoreRead  DataStoreName=workstation_steering
  Data Store Write1 : DataStoreWrite  Commented=on  DataStoreName=Vzuoqian
  Data Store Write2 : DataStoreWrite  Commented=on  DataStoreName=Vyouqian
  Data Store Write3 : DataStoreWrite  Commented=on  DataStoreName=Vzuohou
  Data Store Write4 : DataStoreWrite  Commented=on  DataStoreName=Vyouhou
  LQR差速 : MATLAB Function  TreatAsAtomicUnit=on
  MATLAB Function : MATLAB Function  TreatAsAtomicUnit=on
  Product : Product
  Sum : Sum  Inputs=|+-
  pid : MATLAB Function  Commented=on  TreatAsAtomicUnit=on
  pid1 : MATLAB Function  Commented=on  TreatAsAtomicUnit=on
  pid2 : MATLAB Function  Commented=on  TreatAsAtomicUnit=on
  pid3 : MATLAB Function  Commented=on  TreatAsAtomicUnit=on
  期望横摆力矩计算 : MATLAB Function  TreatAsAtomicUnit=on
  转动惯量 : Constant  Value=145
  阿克曼转向 : MATLAB Function  Commented=on  TreatAsAtomicUnit=on
  M : Outport
  wires:
  Product/1 -> Sum/2
  MATLAB Function/1(y) -> 期望横摆力矩计算/1(delta)
  期望横摆力矩计算/1(Mz) -> Sum/1
  Data Store Read1/1 -> 阿克曼转向/1(v), 期望横摆力矩计算/2(Vx)
  转动惯量/1 -> Product/1, LQR差速/3(J)
  Data Store Read/1 -> MATLAB Function/1(u)
  Sum/1 -> LQR差速/1(yaw_error)
  Data Store Read3/1 -> Product/2, LQR差速/2(yaw_rate)
  阿克曼转向/3(wrl) -> Data Store Write3/1
  Data Store Read4/1 -> pid/1(v)
  Data Store Read7/1 -> pid3/1(v)
  阿克曼转向/2(wfr) -> Data Store Write2/1
  Data Store Read5/1 -> pid1/1(v)
  Data Store Read2/1 -> 阿克曼转向/2(a), 期望横摆力矩计算/3(ax)
  阿克曼转向/1(wfl) -> Data Store Write1/1
  Data Store Read6/1 -> pid2/1(v)
  阿克曼转向/4(wrr) -> Data Store Write4/1
  Data Store Read8/1 -> 阿克曼转向/3(angle)
  LQR差速/1(M) -> M/1

== system finalcode/Subsystem/run/ctrl/Subsystem1/control_strategy/限滑/MPC ==
  右后in : Inport
  左后in : Inport  Port=2
  右前in : Inport  Port=3
  左前in : Inport  Port=4
  MPC : Subsystem
  右后 : Outport
  左后 : Outport  Port=2
  右前 : Outport  Port=3
  左前 : Outport  Port=4
  wires:
  右后in/1 -> MPC/1(U_init)
  左后in/1 -> MPC/2(U_init1)
  右前in/1 -> MPC/3(U_init2)
  左前in/1 -> MPC/4(U_init3)
  MPC/1(右后) -> 右后/1
  MPC/2(左后) -> 左后/1
  MPC/3(右前) -> 右前/1
  MPC/4(左前) -> 左前/1

== system finalcode/Subsystem/run/ctrl/Subsystem1/control_strategy/限滑/PID限滑 ==
  u : Inport
  Constant{,1..3} (4 alike) : Constant  Value=0.9
  Data Store Read : DataStoreRead  DataStoreName=slipyouhou
  Data Store Read1 : DataStoreRead  DataStoreName=slipyuoqian
  Data Store Read2 : DataStoreRead  DataStoreName=slipzuohou
  Data Store Read3 : DataStoreRead  DataStoreName=slipzuoqian
  Data Store Write : DataStoreWrite  DataStoreName=brake_slipyouhou
  Data Store Write1 : DataStoreWrite  DataStoreName=brake_slipzuohou
  Data Store Write2 : DataStoreWrite  DataStoreName=brake_slipzuoqian
  Data Store Write3 : DataStoreWrite  DataStoreName=brake_slipyouqian
  pid限滑与ABS : MATLAB Function  TreatAsAtomicUnit=on
  pid限滑与ABS1 : MATLAB Function  TreatAsAtomicUnit=on
  pid限滑与ABS2 : MATLAB Function  TreatAsAtomicUnit=on
  pid限滑与ABS3 : MATLAB Function  TreatAsAtomicUnit=on
  计算油压 : MATLAB Function  TreatAsAtomicUnit=on
  throttle_youhou : Outport
  throttle_youqian : Outport  Port=2
  throttle_zuohou : Outport  Port=3
  throttle_zuoqian : Outport  Port=4
  wires:
  Data Store Read/1 -> pid限滑与ABS/1(slip)
  Constant/1 -> pid限滑与ABS/2(slip_ratio_limit)
  Data Store Read2/1 -> pid限滑与ABS2/1(slip)
  Constant1/1 -> pid限滑与ABS1/2(slip_ratio_limit)
  Data Store Read3/1 -> pid限滑与ABS3/1(slip)
  pid限滑与ABS/1(throttle) -> throttle_youhou/1
  Constant3/1 -> pid限滑与ABS3/2(slip_ratio_limit)
  Data Store Read1/1 -> pid限滑与ABS1/1(slip)
  Constant2/1 -> pid限滑与ABS2/2(slip_ratio_limit)
  pid限滑与ABS3/1(throttle) -> throttle_zuoqian/1
  pid限滑与ABS1/1(throttle) -> throttle_youqian/1
  pid限滑与ABS2/1(throttle) -> throttle_zuohou/1
  pid限滑与ABS3/2(brake) -> 计算油压/1(y1)
  pid限滑与ABS1/2(brake) -> 计算油压/2(y2)
  pid限滑与ABS2/2(brake) -> 计算油压/3(y3)
  pid限滑与ABS/2(brake) -> 计算油压/4(y4)
  计算油压/4(p4) -> Data Store Write/1
  计算油压/1(p1) -> Data Store Write2/1
  计算油压/2(p2) -> Data Store Write3/1
  计算油压/3(p3) -> Data Store Write1/1
  u/1 -> pid限滑与ABS3/3(u), pid限滑与ABS2/3(u), pid限滑与ABS1/3(u), pid限滑与ABS/3(u)

== system finalcode/Subsystem/run/ctrl/Subsystem1/control_strategy/限滑/Subsystem1 ==
  TP : Inport
  右后 : Inport  Port=2
  throttle_youhou : Inport  Port=3
  In4 : Inport  Port=4
  右前 : Inport  Port=5
  throttle_youqian : Inport  Port=6
  u : Inport  Port=7
  mpc : Inport  Port=8
  pid : Inport  Port=9
  In7 : Inport  Port=10
  左前 : Inport  Port=11
  throttle_zuoqian : Inport  Port=12
  Data Store Read : DataStoreRead  DataStoreName=slipyouhou
  Data Store Read1 : DataStoreRead  DataStoreName=slipyuoqian
  Data Store Read2 : DataStoreRead  DataStoreName=slipzuohou
  Data Store Read3 : DataStoreRead  DataStoreName=slipzuoqian
  Data Store Read4 : DataStoreRead  DataStoreName=match_model
  MATLAB Function2 : MATLAB Function  TreatAsAtomicUnit=on
  MATLAB Function3 : MATLAB Function  TreatAsAtomicUnit=on
  MATLAB Function4 : MATLAB Function  TreatAsAtomicUnit=on
  MATLAB Function5 : MATLAB Function  TreatAsAtomicUnit=on
  youhou : Outport
  youqian : Outport  Port=2
  zuohou : Outport  Port=3
  zuoqian : Outport  Port=4
  wires:
  pid/1 -> MATLAB Function5/3(pid)
  mpc/1 -> MATLAB Function5/2(mpc)
  u/1 -> MATLAB Function5/1(u)
  In4/1 -> MATLAB Function4/1(u)
  右前/1 -> MATLAB Function4/2(mpc)
  throttle_youqian/1 -> MATLAB Function4/3(pid)
  throttle_youhou/1 -> MATLAB Function3/3(pid)
  右后/1 -> MATLAB Function3/2(mpc)
  TP/1 -> MATLAB Function3/1(u)
  throttle_zuoqian/1 -> MATLAB Function2/3(pid)
  左前/1 -> MATLAB Function2/2(mpc)
  In7/1 -> MATLAB Function2/1(u)
  Data Store Read/1 -> MATLAB Function3/4(slip)
  Data Store Read1/1 -> MATLAB Function4/4(slip)
  Data Store Read2/1 -> MATLAB Function5/4(slip)
  Data Store Read3/1 -> MATLAB Function2/4(slip)
  MATLAB Function3/1(y) -> youhou/1
  MATLAB Function2/1(y) -> zuoqian/1
  MATLAB Function5/1(y) -> zuohou/1
  MATLAB Function4/1(y) -> youqian/1
  Data Store Read4/1 -> MATLAB Function2/5(model), MATLAB Function5/5(model), MATLAB Function4/5(model), MATLAB Function3/5(model)

== system finalcode/Subsystem/run/analog_input/无人意图转译/无人/Subsystem1/Desired/Subsystem ==
  y : Inport
  Delay : Delay  DelayLength=1
  Delay1 : Delay
  Delay2 : Delay  DelayLength=3
  Delay3 : Delay  DelayLength=4
  u2 : Outport
  u3 : Outport  Port=2
  u4 : Outport  Port=3
  u5 : Outport  Port=4
  wires:
  y/1 -> Delay3/1, Delay2/1, Delay1/1, Delay/1
  Delay/1 -> u2/1
  Delay1/1 -> u3/1
  Delay3/1 -> u5/1
  Delay2/1 -> u4/1

== system finalcode/Subsystem/run/analog_input/无人意图转译/无人/Subsystem1/Desired/Subsystem1 ==
  y : Inport
  Delay : Delay  DelayLength=1
  Delay1 : Delay
  Delay2 : Delay  DelayLength=3
  Delay3 : Delay  DelayLength=4
  u2 : Outport
  u3 : Outport  Port=2
  u4 : Outport  Port=3
  u5 : Outport  Port=4
  wires:
  y/1 -> Delay3/1, Delay2/1, Delay1/1, Delay/1
  Delay/1 -> u2/1
  Delay1/1 -> u3/1
  Delay3/1 -> u5/1
  Delay2/1 -> u4/1

== system finalcode/Subsystem/run/analog_input/无人意图转译/无人/Subsystem1/进esc控制策略/pid_function ==
  u : Inport
  期望加速度（负值） : Inport  Port=2
  Abs1 : Abs  Commented=on
  Gain : Gain  Commented=on
  Gain2 : Gain  Commented=on
  Subsystem : Subsystem  Commented=on
  integral : MATLAB Function  TreatAsAtomicUnit=on
  output : Outport
  wires:
  integral/1(output) -> output/1
  Gain/1 -> Abs1/1
  u/1 -> integral/1(u)
  Gain2/1 -> Subsystem/1(In1)
  期望加速度（负值）/1 -> integral/2(vd)

== system finalcode/Subsystem/run/ctrl/Subsystem1/control_strategy/限滑/MPC/MPC ==
  U_init : Inport
  U_init1 : Inport  Port=2
  U_init2 : Inport  Port=3
  U_init3 : Inport  Port=4
  Data Store Read : DataStoreRead  DataStoreName=slipyouhou
  Data Store Read1 : DataStoreRead  DataStoreName=slipzuohou
  Data Store Read2 : DataStoreRead  DataStoreName=slipyuoqian
  Data Store Read3 : DataStoreRead  DataStoreName=slipzuoqian
  MATLAB Function : MATLAB Function  TreatAsAtomicUnit=on
  MATLAB Function1 : MATLAB Function  TreatAsAtomicUnit=on
  MATLAB Function2 : MATLAB Function  TreatAsAtomicUnit=on
  MATLAB Function3 : MATLAB Function  TreatAsAtomicUnit=on
  MPC右前 : Subsystem
  MPC右后 : Subsystem
  MPC左前 : Subsystem
  MPC左后 : Subsystem
  右后 : Outport
  左后 : Outport  Port=2
  右前 : Outport  Port=3
  左前 : Outport  Port=4
  wires:
  MPC右前/1(右前) -> 右前/1
  MPC左前/1(左前) -> 左前/1
  MPC右后/1(右后) -> 右后/1
  U_init3/1 -> MPC左前/1(U_init)
  MPC左后/1(左后) -> 左后/1
  U_init1/1 -> MPC左后/1(U_init)
  U_init2/1 -> MPC右前/1(U_init)
  U_init/1 -> MPC右后/1(U_init)
  Data Store Read/1 -> MATLAB Function/1(u)
  MATLAB Function/1(y) -> MPC右后/Enable
  Data Store Read1/1 -> MATLAB Function1/1(u)
  MATLAB Function1/1(y) -> MPC左后/Enable
  Data Store Read2/1 -> MATLAB Function2/1(u)
  MATLAB Function2/1(y) -> MPC右前/Enable
  Data Store Read3/1 -> MATLAB Function3/1(u)
  MATLAB Function3/1(y) -> MPC左前/Enable

== system finalcode/Subsystem/run/analog_input/无人意图转译/无人/Subsystem1/进esc控制策略/pid_function/Subsystem ==
  In1 : Inport
  Constant1 : Constant  Value=0.02
  Delay1 : Delay  DelayLength=1
  Divide1 : Product  Inputs=*/
  Sum4 : Sum  Inputs=|+-
  Out1 : Outport
  wires:
  Divide1/1 -> Out1/1
  Constant1/1 -> Divide1/2
  Sum4/1 -> Divide1/1
  Delay1/1 -> Sum4/2
  In1/1 -> Sum4/1, Delay1/1

== system finalcode/Subsystem/run/ctrl/Subsystem1/control_strategy/限滑/MPC/MPC/MPC右前 ==
  U_init : Inport
  Enable : EnablePort
  Constant : Constant  Value=0.17
  Data Store Read : DataStoreRead  DataStoreName=slipyuoqian
  MPC_function : MATLAB Function  TreatAsAtomicUnit=on
  Sum : Sum  Inputs=|+-
  右前 : Outport
  wires:
  Data Store Read/1 -> Sum/1
  Constant/1 -> Sum/2
  MPC_function/1(u_k) -> 右前/1
  Sum/1 -> MPC_function/1(x_k)
  U_init/1 -> MPC_function/2(U_init)

== system finalcode/Subsystem/run/ctrl/Subsystem1/control_strategy/限滑/MPC/MPC/MPC右后 ==
  U_init : Inport
  Enable : EnablePort
  Constant : Constant  Value=0.17
  Data Store Read : DataStoreRead  DataStoreName=slipyouhou
  MPC_function : MATLAB Function  TreatAsAtomicUnit=on
  Sum : Sum  Inputs=|+-
  右后 : Outport
  wires:
  Data Store Read/1 -> Sum/1
  Constant/1 -> Sum/2
  MPC_function/1(u_k) -> 右后/1
  Sum/1 -> MPC_function/1(x_k)
  U_init/1 -> MPC_function/2(U_init)

== system finalcode/Subsystem/run/ctrl/Subsystem1/control_strategy/限滑/MPC/MPC/MPC左前 ==
  U_init : Inport
  Enable : EnablePort
  Constant : Constant  Value=0.17
  Data Store Read : DataStoreRead  DataStoreName=slipzuoqian
  MPC_function : MATLAB Function  TreatAsAtomicUnit=on
  Sum : Sum  Inputs=|+-
  左前 : Outport
  wires:
  Data Store Read/1 -> Sum/1
  Constant/1 -> Sum/2
  MPC_function/1(u_k) -> 左前/1
  Sum/1 -> MPC_function/1(x_k)
  U_init/1 -> MPC_function/2(U_init)

== system finalcode/Subsystem/run/ctrl/Subsystem1/control_strategy/限滑/MPC/MPC/MPC左后 ==
  U_init : Inport
  Enable : EnablePort
  Constant : Constant  Value=0.17
  Data Store Read : DataStoreRead  DataStoreName=slipzuohou
  MPC_function : MATLAB Function  TreatAsAtomicUnit=on
  Sum : Sum  Inputs=|+-
  左后 : Outport
  wires:
  Data Store Read/1 -> Sum/1
  Constant/1 -> Sum/2
  MPC_function/1(u_k) -> 左后/1
  Sum/1 -> MPC_function/1(x_k)
  U_init/1 -> MPC_function/2(U_init)

== matlab function finalcode/Subsystem/Tx/TX控制器/速度/189左后/MATLAB Function3 ==
  data: v input; y output; angle input; vz input; model input
function y = fcn(v, angle, vz,model)
if (angle>3||angle<-3)&&model==3%4650000,4870000,4741002
    y=vz*594.06;
else
    y = v;
end

== matlab function finalcode/Subsystem/Tx/转向/转向换算/Subsystem/MATLAB Function1 ==
  data: u input; y output
function y = fcn(u)

y = (u-2.846e+04)/3255;

== matlab function finalcode/Subsystem/Tx/TX控制器/Subsystem1/MATLAB Function2 ==
  data: v_guandao input; anglenb input; youqianvvv output; v input; zuoqianvvv output; youhouvvv output; zuohouvvv output; model input; akeman input; kkk input; v_youqian_guandao output; v_youhou_guandao output; v_zuoqian_guandao output; v_zuohou_guandao output
function [youqianvvv,zuoqianvvv,youhouvvv,zuohouvvv,v_youqian_guandao,v_youhou_guandao,v_zuoqian_guandao,v_zuohou_guandao] = fcn( v_guandao, anglenb,v,model,akeman, kkk)
    if kkk==0
         k=-0.05;
     else
        k=kkk;
    end
tg=tan(deg2rad(anglenb))*(1-k);
%Bf=1.18;
%Br=1.16;
Bf=0.93;
Br=1;
L=1.53;%前后轴距

if model==3&&v>3&&anglenb<0
        zuoqianvvv=v*sqrt(tg^2+(1-Bf*tg/(2*L))^2);
        youqianvvv=v*sqrt(tg^2+(1+Bf*tg/(2*L))^2);
        zuohouvvv=v*(1-Br*tg/(2*L));
        youhouvvv=v*(1+Br*tg/(2*L));
elseif model==3&&v>3&&anglenb>0
        zuoqianvvv=v*sqrt(tg^2+(1-Bf*tg/(2*L))^2);
        youqianvvv=v*sqrt(tg^2+(1+Bf*tg/(2*L))^2);
        zuohouvvv=v*(1-Br*tg/(2*L));
        youhouvvv=v*(1+Br*tg/(2*L));    
else
    zuohouvvv=v;
    youhouvvv=v;
    zuoqianvvv=v;
    youqianvvv=v;
end
        v_zuoqian_guandao=v_guandao*sqrt(tg^2+(1-Bf*tg/(2*L))^2);
        v_youqian_guandao=v_guandao*sqrt(tg^2+(1+Bf*tg/(2*L))^2);
        v_zuohou_guandao=v_guandao*(1-Br*tg/(2*L));
        v_youhou_guandao=v_guandao*(1+Br*tg/(2*L));

== matlab function finalcode/转向自动标定/MATLAB Function1 ==
  data: model input; y output; status input
function y = fcn(model,status)
if (model==2)
    y=1;
else
    y=0;
end

== matlab function finalcode/转向自动标定/转向自动标定/MATLAB Function ==
  data: biaozhi1 output
function biaozhi1  = fcn()
persistent i;
     % 初始化状态变量
    if isempty(i)
        i = 1;
    end

    if i>4
        biaozhi1=1;
    else
        biaozhi1=0;       
    end
i=i+1;
end

== matlab function finalcode/转向自动标定/转向自动标定/MATLAB Function1 ==
  data: y1 output; y2 output; biaozhi2 output
function [y1,y2,biaozhi2] = fcn()
    persistent i;
     % 初始化状态变量
    if isempty(i)
        i = 1;
    end
    
    if i<4
        biaozhi2=1;
    else
        biaozhi2=0;
    end
    if mod(i, 2) == 0
        result = 1;
    else
        result = 0;
    end
    
    if result==0
        y1=6307883;
        y2=0;
    else
        y1=6307883;
        y2=128;
    end
    i=i+1;

== matlab function finalcode/Subsystem/Tx/Toworkstation/MATLAB Function ==
  data: u input; y output
function y = fcn(u)
if u~=0&&u~=9&&u~=2
    y=1;
else
    y=0;
end

== matlab function finalcode/Subsystem/Tx/esc，ABS/Subsystem/MATLAB Function ==
  data: u input; y output; status input
function y = fcn(u,status)
y = u;
if status==5
    u=4500;
end

== matlab function finalcode/Subsystem/Tx/esc，ABS/Subsystem/MATLAB Function1 ==
  data: u input; y output; status input
function y = fcn(u,status)
y = u;
if status==5
    u=4500;
end

== matlab function finalcode/Subsystem/Tx/esc，ABS/Subsystem/MATLAB Function2 ==
  data: u input; y output; status input
function y = fcn(u,status)
y = u;
if status==5
    u=4500;
end

== matlab function finalcode/Subsystem/Tx/TX控制器/速度/188右后/MATLAB Function5 ==
  data: v input; y output; angle input; vz input; model input
function y = fcn(v, angle, vz,model)
if(angle>3||angle<-3)&&model==3%4650000,4870000,4741002
    y=vz*594.06;
else
    y = v;
end

== matlab function finalcode/Subsystem/Tx/esc，ABS/Subsystem/MATLAB Function3 ==
  data: u input; y output; status input
function y = fcn(u,status)
y = u;
if status==5
    u=4500;
end
